simulink model "EquationVerifier"  (R2019b)
settings: Solver=VariableStepAuto  StartTime=0.0  StopTime=10.0  RelTol=1e-3
settings Model: Creator=trulsmartinsson  LastModifiedBy=trulsmartinsson

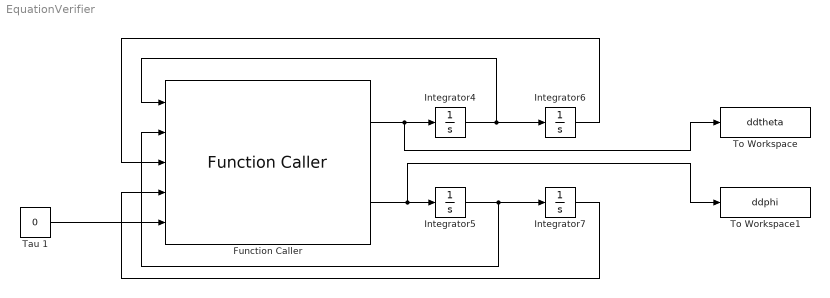
== system EquationVerifier ==
  Function Caller : FunctionCaller  FunctionPrototype=[ddtheta,ddphi] = EqVerify(dtheta,dphi,theta,phi,tau)  InputArgumentSpecifications=<Enter example>  OutputArgumentSpecifications=<Enter example>
  Integrator{4..7} (4 alike) : Integrator
  Tau 1 : Constant  Value=0
  To Workspace : ToWorkspace  VariableName=ddtheta  SaveFormat=Timeseries  SampleTime=-1
  To Workspace1 : ToWorkspace  VariableName=ddphi  SaveFormat=Timeseries  SampleTime=-1
  wires:
  Integrator7/1 -> Function Caller/4
  Integrator5/1 -> Function Caller/2, Integrator7/1
  Integrator4/1 -> Function Caller/1, Integrator6/1
  Tau 1/1 -> Function Caller/5
  Integrator6/1 -> Function Caller/3
  Function Caller/1 -> To Workspace/1, Integrator4/1
  Function Caller/2 -> Integrator5/1, To Workspace1/1
